simulink model "project_2_part2_ex2"  (R2026a)
settings: Solver=VariableStepAuto  StopTime=Tfin
values from neighbouring files (symbols this model uses):
  refPoses = [Xr,Yr,psir]    [part2.m]
  zel = [Xl;Yl;psil;vxl;vyl;wpsil]    [part2.m]
libraries: slpidlib x4
settings Model: Creator=matte  LastModifiedBy=matte
settings ConfigComp: PLC_TargetIDE=codesys35  PLC_MultiTBSigbuilderTimeRange=off  PLC_FoldFBCallOutputVar=off  PLC_RemoveUnusedSSMethodCallArguments=off  PLC_UseCallOutputArgSyntax=off  PLC_EnableUnsignedAndDoubleTypes=off  PLC_EnableUDTSplitting=off  PLC_MaxFieldsInUDT=500.0  PLC_InlineEnumCastFunction=off  PLC_RTWMaxIdLength=31.0  PLC_RollThreshold=5.0  PLC_ActiveTab=0.0  PLC_EnableStringLiteralTB=on  PLC_Enable64bitIntSupport=off

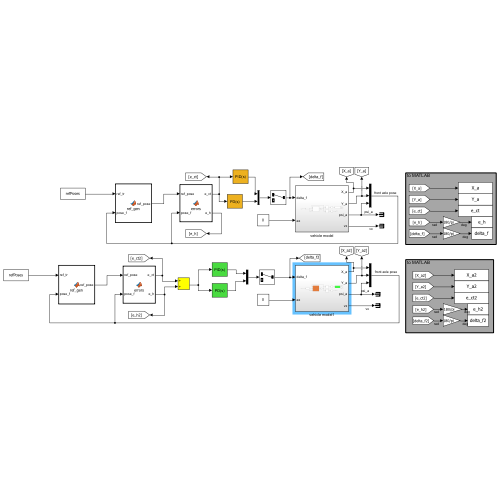
[thumbnail: Simulink's stored preview of the top-level diagram]
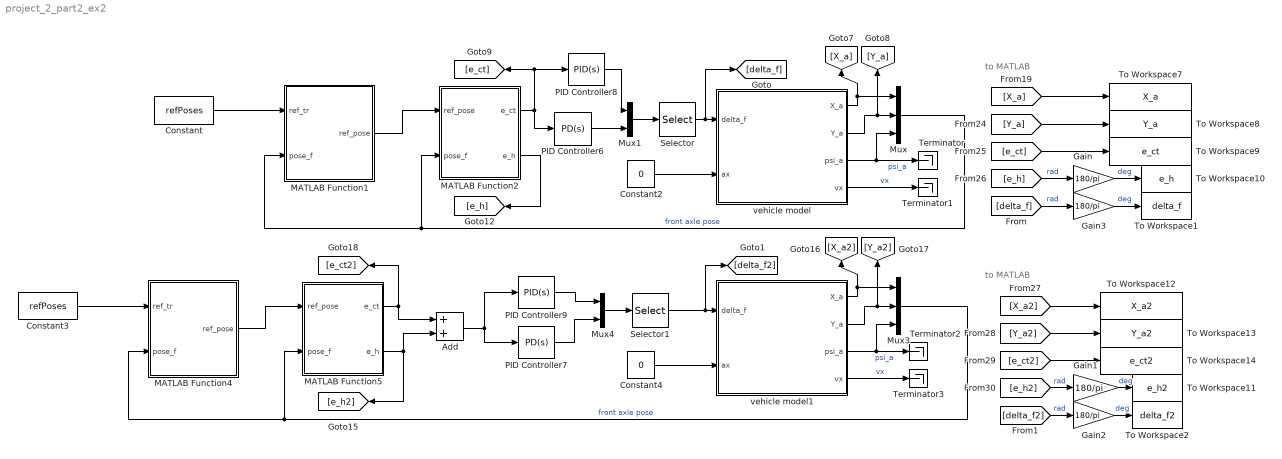
== system project_2_part2_ex2 ==
  note: to MATLAB
  note: to MATLAB
  Add : Sum
  Constant : Constant  Value=refPoses
  Constant2 : Constant  Value=0
  Constant3 : Constant  Value=refPoses
  Constant4 : Constant  Value=0
  Gain{,1..3} (4 alike) : Gain  Gain=180/pi
  MATLAB Function1 : MATLAB Function  TreatAsAtomicUnit=on
  MATLAB Function2 : MATLAB Function  TreatAsAtomicUnit=on  VariantControl=Choice
  MATLAB Function4 : MATLAB Function  TreatAsAtomicUnit=on
  MATLAB Function5 : MATLAB Function  TreatAsAtomicUnit=on  VariantControl=Choice
  Mux : Mux  Inputs=3
  Mux1 : Mux  Inputs=2
  Mux3 : Mux  Inputs=3
  Mux4 : Mux  Inputs=2
  PID Controller6 : slpidlib/PID Controller  Controller=PD  Form=Parallel  TimeDomain=Continuous-time  UseExternalTs=off  SampleTime=-1  IntegratorMethod=Forward Euler  FilterMethod=Forward Euler  ControllerParametersSource=internal  P=0.0293993824477246  I=1  UseKiTs=off  D=0.133630916838169  UseExternalDerivativeSource=off  N=8.1070211736481  UseFilter=on  TunerSelectOption=Transfer Function Based (PID Tuner App)  InitialConditionSource=internal  InitialConditionForIntegrator=0  InitialConditionForFilter=0  DifferentiatorICPrevScaledInput=0  ExternalReset=none  TrackingMode=off  Kt=1  LimitOutput=off  SatLimitsSource=internal  UpperSaturationLimit=inf  LowerSaturationLimit=-inf  LinearizeAsGain=on  AntiWindupMode=none  Kb=1  LimitIntegrator=off  UpperIntegratorSaturationLimit=inf  LowerIntegratorSaturationLimit=-inf  POutMin=[]  POutMax=[]  IOutMin=[]  IOutMax=[]  DOutMin=[]  DOutMax=[]  NOutMin=[]  NOutMax=[]  SumOutMin=[]  SumOutMax=[]  SaturationOutMin=[]  SaturationOutMax=[]  PParamMin=[]  PParamMax=[]  IParamMin=[]  IParamMax=[]  DParamMin=[]  DParamMax=[]  NParamMin=[]  NParamMax=[]  KbParamMin=[]  KbParamMax=[]  KtParamMin=[]  KtParamMax=[]  KbOutMin=[]  KbOutMax=[]  KtOutMin=[]  KtOutMax=[]  IntegratorOutMin=[]  IntegratorOutMax=[]  FilterOutMin=[]  FilterOutMax=[]  SumI1OutMin=[]  SumI1OutMax=[]  SumI2OutMin=[]  SumI2OutMax=[]  SumI3OutMin=[]  SumI3OutMax=[]  SumI4OutMin=[]  SumI4OutMax=[]  SumDOutMin=[]  SumDOutMax=[]  DifferentiatorOutMin=[]  DifferentiatorOutMax=[]  FilterDiffOutCoefMin=[]  FilterDiffOutCoefMax=[]  ReciprocalOutMin=[]  ReciprocalOutMax=[]  SumDenOutMin=[]  SumDenOutMax=[]  SumNumOutMin=[]  SumNumOutMax=[]  DivideOutMin=[]  DivideOutMax=[]  UdiffTsProdOutMin=[]  UdiffTsProdOutMax=[]  NTsProdOutMin=[]  NTsProdOutMax=[]  UintegralTsProdOutMin=[]  UintegralTsProdOutMax=[]  UngainTsProdOutMin=[]  UngainTsProdOutMax=[]  ClampingZeroOutDataTypeStr=Inherit: Inherit via back propagation  ClampingZeroOutMin=[]  ClampingZeroOutMax=[]  FilterDenConstantOutDataTypeStr=Inherit: Inherit via back propagation  FilterDenConstantOutMin=[]  FilterDenConstantOutMax=[]  PCopyOutDataTypeStr=Inherit: Inherit via back propagation  PCopyOutMin=[]  PCopyOutMax=[]  NCopyOutDataTypeStr=Inherit: Inherit via back propagation  NCopyOutMin=[]  NCopyOutMax=[]  IntegratorContinuousStateAttributes=''  IntegratorStateMustResolveToSignalObject=off  IntegratorRTWStateStorageClass=Auto  FilterContinuousStateAttributes=''  FilterStateMustResolveToSignalObject=off  FilterRTWStateStorageClass=Auto  ParallelPVariant=InternalParameters  IdealPVariant=Disabled  IVariant=Disabled  DVariant=InternalParameters  IntegratorVariant=Disabled  SatVariant=Disabled  AWVariant=Disabled  PCopyVariant=Disabled  TRVariant=Disabled  FdbkBlocksVariant=Forward  IdealPFdbkVariant=Disabled  SatFdbkVariant=Disabled  DerivativeFilterVariant=ContFilter  NVariant=InternalParameters  NCopyVariant=Disabled  FilterICVariant=InternalICsFilter  IntegratorICVariant=Disabled  ExternalResetVariant=Disabled  TRSumVariant=Passthrough  SumFdbkVariant=Disabled  SumVariant=Sum_PD  TsampFilterVariant=InternalTs  TsampNgainVariant=Passthrough  TsampIntegralVariant=Disabled_SignalSpec  ExternalSaturationOutDataTypeStr=Inherit: Same as second input  DerivativeSourceVariant=ErrorSignal  PreIntVariant=InternalPreInt
  PID Controller7 : slpidlib/PID Controller  Controller=PD  Form=Parallel  TimeDomain=Continuous-time  UseExternalTs=off  SampleTime=-1  IntegratorMethod=Forward Euler  FilterMethod=Forward Euler  ControllerParametersSource=internal  P=0.0228533895273018  I=1  UseKiTs=off  D=0.0667779764282045  UseExternalDerivativeSource=off  N=10.5082235429226  UseFilter=on  TunerSelectOption=Transfer Function Based (PID Tuner App)  InitialConditionSource=internal  InitialConditionForIntegrator=0  InitialConditionForFilter=0  DifferentiatorICPrevScaledInput=0  ExternalReset=none  TrackingMode=off  Kt=1  LimitOutput=off  SatLimitsSource=internal  UpperSaturationLimit=inf  LowerSaturationLimit=-inf  LinearizeAsGain=on  AntiWindupMode=none  Kb=1  LimitIntegrator=off  UpperIntegratorSaturationLimit=inf  LowerIntegratorSaturationLimit=-inf  POutMin=[]  POutMax=[]  IOutMin=[]  IOutMax=[]  DOutMin=[]  DOutMax=[]  NOutMin=[]  NOutMax=[]  SumOutMin=[]  SumOutMax=[]  SaturationOutMin=[]  SaturationOutMax=[]  PParamMin=[]  PParamMax=[]  IParamMin=[]  IParamMax=[]  DParamMin=[]  DParamMax=[]  NParamMin=[]  NParamMax=[]  KbParamMin=[]  KbParamMax=[]  KtParamMin=[]  KtParamMax=[]  KbOutMin=[]  KbOutMax=[]  KtOutMin=[]  KtOutMax=[]  IntegratorOutMin=[]  IntegratorOutMax=[]  FilterOutMin=[]  FilterOutMax=[]  SumI1OutMin=[]  SumI1OutMax=[]  SumI2OutMin=[]  SumI2OutMax=[]  SumI3OutMin=[]  SumI3OutMax=[]  SumI4OutMin=[]  SumI4OutMax=[]  SumDOutMin=[]  SumDOutMax=[]  DifferentiatorOutMin=[]  DifferentiatorOutMax=[]  FilterDiffOutCoefMin=[]  FilterDiffOutCoefMax=[]  ReciprocalOutMin=[]  ReciprocalOutMax=[]  SumDenOutMin=[]  SumDenOutMax=[]  SumNumOutMin=[]  SumNumOutMax=[]  DivideOutMin=[]  DivideOutMax=[]  UdiffTsProdOutMin=[]  UdiffTsProdOutMax=[]  NTsProdOutMin=[]  NTsProdOutMax=[]  UintegralTsProdOutMin=[]  UintegralTsProdOutMax=[]  UngainTsProdOutMin=[]  UngainTsProdOutMax=[]  ClampingZeroOutDataTypeStr=Inherit: Inherit via back propagation  ClampingZeroOutMin=[]  ClampingZeroOutMax=[]  FilterDenConstantOutDataTypeStr=Inherit: Inherit via back propagation  FilterDenConstantOutMin=[]  FilterDenConstantOutMax=[]  PCopyOutDataTypeStr=Inherit: Inherit via back propagation  PCopyOutMin=[]  PCopyOutMax=[]  NCopyOutDataTypeStr=Inherit: Inherit via back propagation  NCopyOutMin=[]  NCopyOutMax=[]  IntegratorContinuousStateAttributes=''  IntegratorStateMustResolveToSignalObject=off  IntegratorRTWStateStorageClass=Auto  FilterContinuousStateAttributes=''  FilterStateMustResolveToSignalObject=off  FilterRTWStateStorageClass=Auto  ParallelPVariant=InternalParameters  IdealPVariant=Disabled  IVariant=Disabled  DVariant=InternalParameters  IntegratorVariant=Disabled  SatVariant=Disabled  AWVariant=Disabled  PCopyVariant=Disabled  TRVariant=Disabled  FdbkBlocksVariant=Forward  IdealPFdbkVariant=Disabled  SatFdbkVariant=Disabled  DerivativeFilterVariant=ContFilter  NVariant=InternalParameters  NCopyVariant=Disabled  FilterICVariant=InternalICsFilter  IntegratorICVariant=Disabled  ExternalResetVariant=Disabled  TRSumVariant=Passthrough  SumFdbkVariant=Disabled  SumVariant=Sum_PD  TsampFilterVariant=InternalTs  TsampNgainVariant=Passthrough  TsampIntegralVariant=Disabled_SignalSpec  ExternalSaturationOutDataTypeStr=Inherit: Same as second input  DerivativeSourceVariant=ErrorSignal  PreIntVariant=InternalPreInt
  PID Controller8 : slpidlib/PID Controller  Controller=PID  Form=Parallel  TimeDomain=Continuous-time  UseExternalTs=off  SampleTime=-1  IntegratorMethod=Forward Euler  FilterMethod=Forward Euler  ControllerParametersSource=internal  P=0.12886307975281  I=0.00700241271226333  UseKiTs=off  D=0.240534845983153  UseExternalDerivativeSource=off  N=9.98423320623587  UseFilter=on  TunerSelectOption=Transfer Function Based (PID Tuner App)  InitialConditionSource=internal  InitialConditionForIntegrator=0  InitialConditionForFilter=0  DifferentiatorICPrevScaledInput=0  ExternalReset=none  TrackingMode=off  Kt=1  LimitOutput=off  SatLimitsSource=internal  UpperSaturationLimit=inf  LowerSaturationLimit=-inf  LinearizeAsGain=on  AntiWindupMode=none  Kb=1  LimitIntegrator=off  UpperIntegratorSaturationLimit=inf  LowerIntegratorSaturationLimit=-inf  POutMin=[]  POutMax=[]  IOutMin=[]  IOutMax=[]  DOutMin=[]  DOutMax=[]  NOutMin=[]  NOutMax=[]  SumOutMin=[]  SumOutMax=[]  SaturationOutMin=[]  SaturationOutMax=[]  PParamMin=[]  PParamMax=[]  IParamMin=[]  IParamMax=[]  DParamMin=[]  DParamMax=[]  NParamMin=[]  NParamMax=[]  KbParamMin=[]  KbParamMax=[]  KtParamMin=[]  KtParamMax=[]  KbOutMin=[]  KbOutMax=[]  KtOutMin=[]  KtOutMax=[]  IntegratorOutMin=[]  IntegratorOutMax=[]  FilterOutMin=[]  FilterOutMax=[]  SumI1OutMin=[]  SumI1OutMax=[]  SumI2OutMin=[]  SumI2OutMax=[]  SumI3OutMin=[]  SumI3OutMax=[]  SumI4OutMin=[]  SumI4OutMax=[]  SumDOutMin=[]  SumDOutMax=[]  DifferentiatorOutMin=[]  DifferentiatorOutMax=[]  FilterDiffOutCoefMin=[]  FilterDiffOutCoefMax=[]  ReciprocalOutMin=[]  ReciprocalOutMax=[]  SumDenOutMin=[]  SumDenOutMax=[]  SumNumOutMin=[]  SumNumOutMax=[]  DivideOutMin=[]  DivideOutMax=[]  UdiffTsProdOutMin=[]  UdiffTsProdOutMax=[]  NTsProdOutMin=[]  NTsProdOutMax=[]  UintegralTsProdOutMin=[]  UintegralTsProdOutMax=[]  UngainTsProdOutMin=[]  UngainTsProdOutMax=[]  ClampingZeroOutDataTypeStr=Inherit: Inherit via back propagation  ClampingZeroOutMin=[]  ClampingZeroOutMax=[]  FilterDenConstantOutDataTypeStr=Inherit: Inherit via back propagation  FilterDenConstantOutMin=[]  FilterDenConstantOutMax=[]  PCopyOutDataTypeStr=Inherit: Inherit via back propagation  PCopyOutMin=[]  PCopyOutMax=[]  NCopyOutDataTypeStr=Inherit: Inherit via back propagation  NCopyOutMin=[]  NCopyOutMax=[]  IntegratorContinuousStateAttributes=''  IntegratorStateMustResolveToSignalObject=off  IntegratorRTWStateStorageClass=Auto  FilterContinuousStateAttributes=''  FilterStateMustResolveToSignalObject=off  FilterRTWStateStorageClass=Auto  ParallelPVariant=InternalParameters  IdealPVariant=Disabled  IVariant=InternalParameters  DVariant=InternalParameters  IntegratorVariant=Continuous  SatVariant=Disabled  AWVariant=Passthrough  PCopyVariant=Disabled  TRVariant=Disabled  FdbkBlocksVariant=Forward  IdealPFdbkVariant=Disabled  SatFdbkVariant=Disabled  DerivativeFilterVariant=ContFilter  NVariant=InternalParameters  NCopyVariant=Disabled  FilterICVariant=InternalICsFilter  IntegratorICVariant=InternalICs  ExternalResetVariant=Disabled  TRSumVariant=Passthrough  SumFdbkVariant=Disabled  SumVariant=Sum_PID  TsampFilterVariant=InternalTs  TsampNgainVariant=Passthrough  TsampIntegralVariant=Disabled_SignalSpec  ExternalSaturationOutDataTypeStr=Inherit: Same as second input  DerivativeSourceVariant=ErrorSignal  PreIntVariant=InternalPreInt
  PID Controller9 : slpidlib/PID Controller  Controller=PID  Form=Parallel  TimeDomain=Continuous-time  UseExternalTs=off  SampleTime=-1  IntegratorMethod=Forward Euler  FilterMethod=Forward Euler  ControllerParametersSource=internal  P=0.06842463877229  I=0.0106232727854251  UseKiTs=off  D=0.102172985034677  UseExternalDerivativeSource=off  N=8.201434209133  UseFilter=on  TunerSelectOption=Transfer Function Based (PID Tuner App)  InitialConditionSource=internal  InitialConditionForIntegrator=0  InitialConditionForFilter=0  DifferentiatorICPrevScaledInput=0  ExternalReset=none  TrackingMode=off  Kt=1  LimitOutput=off  SatLimitsSource=internal  UpperSaturationLimit=inf  LowerSaturationLimit=-inf  LinearizeAsGain=on  AntiWindupMode=none  Kb=1  LimitIntegrator=off  UpperIntegratorSaturationLimit=inf  LowerIntegratorSaturationLimit=-inf  POutMin=[]  POutMax=[]  IOutMin=[]  IOutMax=[]  DOutMin=[]  DOutMax=[]  NOutMin=[]  NOutMax=[]  SumOutMin=[]  SumOutMax=[]  SaturationOutMin=[]  SaturationOutMax=[]  PParamMin=[]  PParamMax=[]  IParamMin=[]  IParamMax=[]  DParamMin=[]  DParamMax=[]  NParamMin=[]  NParamMax=[]  KbParamMin=[]  KbParamMax=[]  KtParamMin=[]  KtParamMax=[]  KbOutMin=[]  KbOutMax=[]  KtOutMin=[]  KtOutMax=[]  IntegratorOutMin=[]  IntegratorOutMax=[]  FilterOutMin=[]  FilterOutMax=[]  SumI1OutMin=[]  SumI1OutMax=[]  SumI2OutMin=[]  SumI2OutMax=[]  SumI3OutMin=[]  SumI3OutMax=[]  SumI4OutMin=[]  SumI4OutMax=[]  SumDOutMin=[]  SumDOutMax=[]  DifferentiatorOutMin=[]  DifferentiatorOutMax=[]  FilterDiffOutCoefMin=[]  FilterDiffOutCoefMax=[]  ReciprocalOutMin=[]  ReciprocalOutMax=[]  SumDenOutMin=[]  SumDenOutMax=[]  SumNumOutMin=[]  SumNumOutMax=[]  DivideOutMin=[]  DivideOutMax=[]  UdiffTsProdOutMin=[]  UdiffTsProdOutMax=[]  NTsProdOutMin=[]  NTsProdOutMax=[]  UintegralTsProdOutMin=[]  UintegralTsProdOutMax=[]  UngainTsProdOutMin=[]  UngainTsProdOutMax=[]  ClampingZeroOutDataTypeStr=Inherit: Inherit via back propagation  ClampingZeroOutMin=[]  ClampingZeroOutMax=[]  FilterDenConstantOutDataTypeStr=Inherit: Inherit via back propagation  FilterDenConstantOutMin=[]  FilterDenConstantOutMax=[]  PCopyOutDataTypeStr=Inherit: Inherit via back propagation  PCopyOutMin=[]  PCopyOutMax=[]  NCopyOutDataTypeStr=Inherit: Inherit via back propagation  NCopyOutMin=[]  NCopyOutMax=[]  IntegratorContinuousStateAttributes=''  IntegratorStateMustResolveToSignalObject=off  IntegratorRTWStateStorageClass=Auto  FilterContinuousStateAttributes=''  FilterStateMustResolveToSignalObject=off  FilterRTWStateStorageClass=Auto  ParallelPVariant=InternalParameters  IdealPVariant=Disabled  IVariant=InternalParameters  DVariant=InternalParameters  IntegratorVariant=Continuous  SatVariant=Disabled  AWVariant=Passthrough  PCopyVariant=Disabled  TRVariant=Disabled  FdbkBlocksVariant=Forward  IdealPFdbkVariant=Disabled  SatFdbkVariant=Disabled  DerivativeFilterVariant=ContFilter  NVariant=InternalParameters  NCopyVariant=Disabled  FilterICVariant=InternalICsFilter  IntegratorICVariant=InternalICs  ExternalResetVariant=Disabled  TRSumVariant=Passthrough  SumFdbkVariant=Disabled  SumVariant=Sum_PID  TsampFilterVariant=InternalTs  TsampNgainVariant=Passthrough  TsampIntegralVariant=Disabled_SignalSpec  ExternalSaturationOutDataTypeStr=Inherit: Same as second input  DerivativeSourceVariant=ErrorSignal  PreIntVariant=InternalPreInt
  Selector : Selector  InputPortWidth=2  IndexOptions=Index vector (dialog)  Indices=controller1  OutputSizes=1  RuntimeRangeChecks=on
  Selector1 : Selector  InputPortWidth=2  IndexOptions=Index vector (dialog)  Indices=controller2  OutputSizes=1  RuntimeRangeChecks=on
  Terminator{,1..3} (4 alike) : Terminator
  To Workspace1 : ToWorkspace  VariableName=delta_f  SaveFormat=Timeseries  SampleTime=-1
  To Workspace10 : ToWorkspace  VariableName=e_h  SaveFormat=Timeseries  SampleTime=-1
  To Workspace11 : ToWorkspace  VariableName=e_h2  SaveFormat=Timeseries  SampleTime=-1
  To Workspace12 : ToWorkspace  VariableName=X_a2  SaveFormat=Timeseries  SampleTime=-1
  To Workspace13 : ToWorkspace  VariableName=Y_a2  SaveFormat=Timeseries  SampleTime=-1
  To Workspace14 : ToWorkspace  VariableName=e_ct2  SaveFormat=Timeseries  SampleTime=-1
  To Workspace2 : ToWorkspace  VariableName=delta_f2  SaveFormat=Timeseries  SampleTime=-1
  To Workspace7 : ToWorkspace  VariableName=X_a  SaveFormat=Timeseries  SampleTime=-1
  To Workspace8 : ToWorkspace  VariableName=Y_a  SaveFormat=Timeseries  SampleTime=-1
  To Workspace9 : ToWorkspace  VariableName=e_ct  SaveFormat=Timeseries  SampleTime=-1
  vehicle model : Subsystem
  vehicle model1 : Subsystem
  wires:
  Constant3/1 -> MATLAB Function4/1(ref_tr)
  vehicle model1/4(vx) -> Terminator3/1  "vx"
  Mux1/1 -> Selector/1
  MATLAB Function5/2(e_h) -> [e_h2], Add/2
  MATLAB Function2/2(e_h) -> [e_h]
  Constant2/1 -> vehicle model/2(ax)
  vehicle model1/1(X_a) -> [X_a2], Mux3/1
  MATLAB Function4/1(ref_pose) -> MATLAB Function5/1(ref_pose)
  MATLAB Function1/1(ref_pose) -> MATLAB Function2/1(ref_pose)
  Constant/1 -> MATLAB Function1/1(ref_tr)
  [X_a2] -> To Workspace12/1
  [e_ct2] -> To Workspace14/1
  [e_ct] -> To Workspace9/1
  vehicle model1/2(Y_a) -> [Y_a2], Mux3/2
  PID Controller9/1 -> Mux4/1
  PID Controller7/1 -> Mux4/2
  [Y_a2] -> To Workspace13/1
  [Y_a] -> To Workspace8/1
  vehicle model/3(psi_a) -> Terminator/1, Mux/3  "psi_a"
  Mux/1 -> MATLAB Function1/2(pose_f), MATLAB Function2/2(pose_f)  "front axle pose"
  Mux3/1 -> MATLAB Function5/2(pose_f), MATLAB Function4/2(pose_f)  "front axle pose"
  PID Controller6/1 -> Mux1/2
  Constant4/1 -> vehicle model1/2(ax)
  MATLAB Function5/1(e_ct) -> Add/1, [e_ct2]
  vehicle model/1(X_a) -> Mux/1, [X_a]
  Add/1 -> PID Controller7/1, PID Controller9/1
  vehicle model/2(Y_a) -> Mux/2, [Y_a]
  Selector1/1 -> [delta_f2], vehicle model1/1(delta_f)
  vehicle model/4(vx) -> Terminator1/1  "vx"
  vehicle model1/3(psi_a) -> Terminator2/1, Mux3/3  "psi_a"
  [X_a] -> To Workspace7/1
  MATLAB Function2/1(e_ct) -> PID Controller6/1, PID Controller8/1, [e_ct]
  PID Controller8/1 -> Mux1/1
  Mux4/1 -> Selector1/1
  Selector/1 -> [delta_f], vehicle model/1(delta_f)
  [delta_f] -> Gain3/1  "rad"
  [delta_f2] -> Gain2/1  "rad"
  [e_h] -> Gain/1  "rad"
  Gain/1 -> To Workspace10/1  "deg"
  [e_h2] -> Gain1/1  "rad"
  Gain1/1 -> To Workspace11/1  "deg"
  Gain2/1 -> To Workspace2/1  "deg"
  Gain3/1 -> To Workspace1/1  "deg"

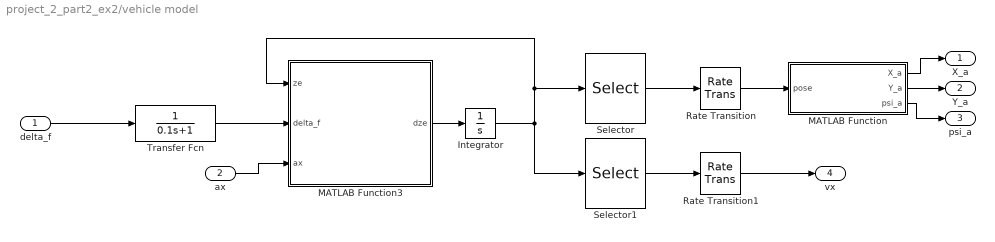
== system project_2_part2_ex2/vehicle model ==
  delta_f : Inport
  ax : Inport  Port=2
  Integrator : Integrator  InitialCondition=zel
  MATLAB Function : MATLAB Function  TreatAsAtomicUnit=on
  MATLAB Function3 : MATLAB Function  TreatAsAtomicUnit=on
  Rate Transition : RateTransition
  Rate Transition1 : RateTransition
  Selector : Selector  InputPortWidth=6  IndexOptions=Index vector (dialog)  Indices=[1:3]  OutputSizes=1
  Selector1 : Selector  InputPortWidth=6  IndexOptions=Index vector (dialog)  Indices=4  OutputSizes=1
  Transfer Fcn : TransferFcn  Denominator=[0.1 1]
  X_a : Outport
  Y_a : Outport  Port=2
  psi_a : Outport  Port=3
  vx : Outport  Port=4
  wires:
  ax/1 -> MATLAB Function3/3(ax)
  MATLAB Function3/1(dze) -> Integrator/1
  Integrator/1 -> MATLAB Function3/1(ze), Selector/1, Selector1/1
  Transfer Fcn/1 -> MATLAB Function3/2(delta_f)
  delta_f/1 -> Transfer Fcn/1
  Selector/1 -> Rate Transition/1
  MATLAB Function/1(X_a) -> X_a/1
  Rate Transition/1 -> MATLAB Function/1(pose)
  Selector1/1 -> Rate Transition1/1
  Rate Transition1/1 -> vx/1
  MATLAB Function/2(Y_a) -> Y_a/1
  MATLAB Function/3(psi_a) -> psi_a/1

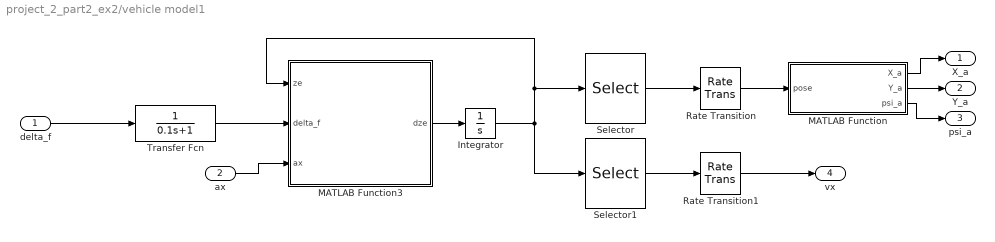
== system project_2_part2_ex2/vehicle model1 ==
  delta_f : Inport
  ax : Inport  Port=2
  Integrator : Integrator  InitialCondition=zel
  MATLAB Function : MATLAB Function  TreatAsAtomicUnit=on
  MATLAB Function3 : MATLAB Function  TreatAsAtomicUnit=on
  Rate Transition : RateTransition
  Rate Transition1 : RateTransition
  Selector : Selector  InputPortWidth=6  IndexOptions=Index vector (dialog)  Indices=[1:3]  OutputSizes=1
  Selector1 : Selector  InputPortWidth=6  IndexOptions=Index vector (dialog)  Indices=4  OutputSizes=1
  Transfer Fcn : TransferFcn  Denominator=[0.1 1]
  X_a : Outport
  Y_a : Outport  Port=2
  psi_a : Outport  Port=3
  vx : Outport  Port=4
  wires:
  MATLAB Function/3(psi_a) -> psi_a/1
  MATLAB Function/2(Y_a) -> Y_a/1
  Rate Transition1/1 -> vx/1
  Selector1/1 -> Rate Transition1/1
  Rate Transition/1 -> MATLAB Function/1(pose)
  MATLAB Function/1(X_a) -> X_a/1
  Selector/1 -> Rate Transition/1
  delta_f/1 -> Transfer Fcn/1
  Transfer Fcn/1 -> MATLAB Function3/2(delta_f)
  Integrator/1 -> Selector1/1, Selector/1, MATLAB Function3/1(ze)
  MATLAB Function3/1(dze) -> Integrator/1
  ax/1 -> MATLAB Function3/3(ax)

== matlab function project_2_part2_ex2/MATLAB Function4 ==
  data: ref_tr input; ref_pose output; pose_f input
function ref_pose=ref_gen(ref_tr,pose_f)

N=size(ref_tr,1);

% reference trajectory closest point to the vehicle
dis=vecnorm(ref_tr(:,1:2)'-pose_f(1:2)*ones(1,N));
[~,c]=min(dis);
ref_pose=ref_tr(c,:)';

end

== matlab function project_2_part2_ex2/MATLAB Function2 ==
  data: ref_pose input; e_ct output; pose_f input; e_h output
function [e_ct,e_h]=errors(ref_pose,pose_f)

% Wrap angles in the interval [0,2*pi]
ref_pose(3)=wrap_to_2pi(ref_pose(3));
pose_f(3)=wrap_to_2pi(pose_f(3));

% Cross-track error  
d=ref_pose(1:2)-pose_f(1:2);
e_ct=d(2)*cos(ref_pose(3))-d(1)*sin(ref_pose(3));

% Heading error
e_h=wrap_to_pi(ref_pose(3)-pose_f(3));

end

%--------------------------------------------------------------------------

function lambda = wrap_to_2pi(lambda)
%   Wraps angle in radians to [0 2*pi]
%   lambdaWrapped = wrapTo2Pi(LAMBDA) wraps angles in LAMBDA, in radians,
%   to the interval [0 2*pi] such that zero maps to zero and 2*pi maps
%   to 2*pi. (In general, positive multiples of 2*pi map to 2*pi and
%   negative multiples of 2*pi map to zero.)
%   See also wrapToPi, wrapTo180, wrapTo360.
positiveInput = (lambda > 0);
lambda = mod(lambda, 2*pi);
lambda((lambda == 0) & positiveInput) = 2*pi;
end

function lambda = wrap_to_pi(lambda)
%   Wraps angle in radians to [-pi pi]
%   lambdaWrapped = wrapToPi(LAMBDA) wraps angles in LAMBDA, in radians,
%   to the interval [-pi pi] such that pi maps to pi and -pi maps to
%   -pi.  (In general, odd, positive multiples of pi map to pi and odd,
%   negative multiples of pi map to -pi.)
%   See also wrapTo2Pi, wrapTo180, wrapTo360.
q = (lambda < -pi) | (pi < lambda);
lambda(q) = wrap_to_2pi(lambda(q) + pi) - pi;
end

== matlab function project_2_part2_ex2/MATLAB Function1 ==
  data: ref_tr input; ref_pose output; pose_f input
function ref_pose=ref_gen(ref_tr,pose_f)

N=size(ref_tr,1);

% reference trajectory closest point to the vehicle
dis=vecnorm(ref_tr(:,1:2)'-pose_f(1:2)*ones(1,N));
[~,c]=min(dis);
ref_pose=ref_tr(c,:)';

end

== matlab function project_2_part2_ex2/vehicle model/MATLAB Function3 ==
  data: ze input; delta_f input; dze output; ax input
function dze = DSTP_nonlinear_model(ze,delta_f, ax)

% States
X = ze(1);
Y =ze(2);
psi = ze(3);
vx = ze(4);
vy = ze(5);
wpsi = ze(6);

% % Inputs
% ax    = u(1);
% delta_f = u(2);

% Vehicle parameters:
l1 = 1.2;       % m
l2 = 1.6;       % m
m = 1575;       % kg
Jz = 4000;      % kg*m^2
C1 = 27e3;      % N/rad
C2 = C1;

% Slip angles (non-linear model)
alpha1 = atan((vy + l1*wpsi)/vx) - delta_f;
alpha2 = atan((vy - l2*wpsi)/vx);

% Pacejka's tire model
[fp_alpha1, fp_alpha2] = pacejka_model(alpha1,alpha2,C1,C2);
Fy1 = -fp_alpha1 * cos(delta_f);
Fy2 = -fp_alpha2;

% State equations
dX    = vx*cos(psi) - vy*sin(psi);
dY    = vx*sin(psi) + vy*cos(psi);
dpsi  = wpsi;
dvx   = vy*wpsi + ax;
dvy   = -vx*wpsi + (2/m)*(Fy1 + Fy2);
dwpsi = (2/Jz)*(l1*Fy1 - l2*Fy2);

dze = [dX; dY; dpsi; dvx; dvy; dwpsi];

% Pacejka Lateral tire forces 
function [fp_alpha1, fp_alpha2] = pacejka_model(alpha1,alpha2,C1,C2)

% Tire parameters:
p1 = 3863;      % N
p2 = 1.5;
p4 = -0.5;
p3_front = C1/p1/p2;  % front tire
p3_rear = C2/p1/p2;   % rear tire

fp_alpha1 = p1*sin(p2*atan(p3_front*alpha1 - p4*(p3_front*alpha1 - atan(p3_front*alpha1))));
fp_alpha2 = p1*sin(p2*atan(p3_rear*alpha2 - p4*(p3_rear*alpha2 - atan(p3_rear*alpha2))));

end
end

== matlab function project_2_part2_ex2/vehicle model/MATLAB Function ==
  data: pose input; X_a output; Y_a output; psi_a output
function [X_a,Y_a,psi_a] = translatePose(pose)
% Parameters
l1 = 1.2;       % m
X_CoG = pose(1);
Y_CoG = pose(2);
psi = pose(3);

% Front axle position
X_a = X_CoG + l1*cos(psi);
Y_a = Y_CoG + l1*sin(psi);
psi_a = psi;
end

== matlab function project_2_part2_ex2/MATLAB Function5 ==
  data: ref_pose input; e_ct output; pose_f input; e_h output
function [e_ct,e_h]=errors(ref_pose,pose_f)

% Wrap angles in the interval [0,2*pi]
ref_pose(3)=wrap_to_2pi(ref_pose(3));
pose_f(3)=wrap_to_2pi(pose_f(3));

% Cross-track error  
d=ref_pose(1:2)-pose_f(1:2);
e_ct=d(2)*cos(ref_pose(3))-d(1)*sin(ref_pose(3));

% Heading error
e_h=wrap_to_pi(ref_pose(3)-pose_f(3));

end

%--------------------------------------------------------------------------

function lambda = wrap_to_2pi(lambda)
%   Wraps angle in radians to [0 2*pi]
%   lambdaWrapped = wrapTo2Pi(LAMBDA) wraps angles in LAMBDA, in radians,
%   to the interval [0 2*pi] such that zero maps to zero and 2*pi maps
%   to 2*pi. (In general, positive multiples of 2*pi map to 2*pi and
%   negative multiples of 2*pi map to zero.)
%   See also wrapToPi, wrapTo180, wrapTo360.
positiveInput = (lambda > 0);
lambda = mod(lambda, 2*pi);
lambda((lambda == 0) & positiveInput) = 2*pi;
end

function lambda = wrap_to_pi(lambda)
%   Wraps angle in radians to [-pi pi]
%   lambdaWrapped = wrapToPi(LAMBDA) wraps angles in LAMBDA, in radians,
%   to the interval [-pi pi] such that pi maps to pi and -pi maps to
%   -pi.  (In general, odd, positive multiples of pi map to pi and odd,
%   negative multiples of pi map to -pi.)
%   See also wrapTo2Pi, wrapTo180, wrapTo360.
q = (lambda < -pi) | (pi < lambda);
lambda(q) = wrap_to_2pi(lambda(q) + pi) - pi;
end

== matlab function project_2_part2_ex2/vehicle model1/MATLAB Function ==
  data: pose input; X_a output; Y_a output; psi_a output
function [X_a,Y_a,psi_a] = translatePose(pose)
% Parameters
l1 = 1.2;       % m
X_CoG = pose(1);
Y_CoG = pose(2);
psi = pose(3);

% Front axle position
X_a = X_CoG + l1*cos(psi);
Y_a = Y_CoG + l1*sin(psi);
psi_a = psi;
end

== matlab function project_2_part2_ex2/vehicle model1/MATLAB Function3 ==
  data: ze input; delta_f input; dze output; ax input
function dze = DSTP_nonlinear_model(ze,delta_f, ax)

% States
X = ze(1);
Y =ze(2);
psi = ze(3);
vx = ze(4);
vy = ze(5);
wpsi = ze(6);

% % Inputs
% ax    = u(1);
% delta_f = u(2);

% Vehicle parameters:
l1 = 1.2;       % m
l2 = 1.6;       % m
m = 1575;       % kg
Jz = 4000;      % kg*m^2
C1 = 27e3;      % N/rad
C2 = C1;

% Slip angles (non-linear model)
alpha1 = atan((vy + l1*wpsi)/vx) - delta_f;
alpha2 = atan((vy - l2*wpsi)/vx);

% Pacejka's tire model
[fp_alpha1, fp_alpha2] = pacejka_model(alpha1,alpha2,C1,C2);
Fy1 = -fp_alpha1 * cos(delta_f);
Fy2 = -fp_alpha2;

% State equations
dX    = vx*cos(psi) - vy*sin(psi);
dY    = vx*sin(psi) + vy*cos(psi);
dpsi  = wpsi;
dvx   = vy*wpsi + ax;
dvy   = -vx*wpsi + (2/m)*(Fy1 + Fy2);
dwpsi = (2/Jz)*(l1*Fy1 - l2*Fy2);

dze = [dX; dY; dpsi; dvx; dvy; dwpsi];

% Pacejka Lateral tire forces 
function [fp_alpha1, fp_alpha2] = pacejka_model(alpha1,alpha2,C1,C2)

% Tire parameters:
p1 = 3863;      % N
p2 = 1.5;
p4 = -0.5;
p3_front = C1/p1/p2;  % front tire
p3_rear = C2/p1/p2;   % rear tire

fp_alpha1 = p1*sin(p2*atan(p3_front*alpha1 - p4*(p3_front*alpha1 - atan(p3_front*alpha1))));
fp_alpha2 = p1*sin(p2*atan(p3_rear*alpha2 - p4*(p3_rear*alpha2 - atan(p3_rear*alpha2))));

end
end
